simulink model "modelReferenceTest"  (Simulink 7.6)
settings: Solver=FixedStepDiscrete  StartTime=0.0  StopTime=10.0  FixedStep=1  RelTol=1e-3
settings Model: Creator=c2wt  LastModifiedBy=c2wt

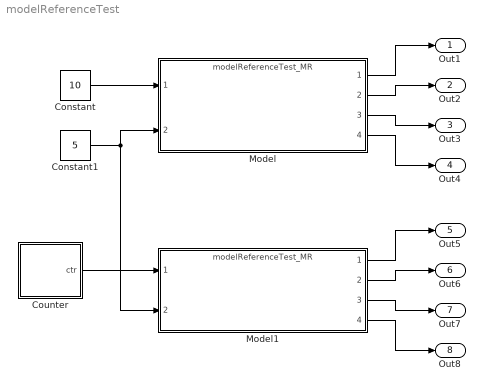
== system modelReferenceTest ==
  Constant : Constant  Value=10
  Constant1 : Constant  Value=5
  Counter : Stateflow chart  TreatAsAtomicUnit=on
  Model : ModelReference  ModelNameDialog=modelReferenceTest_MR  SimulationMode=Accelerator  ModelReferenceVersion=1.4  CopyOfModelName=modelReferenceTest_MR
  Model1 : ModelReference  ModelNameDialog=modelReferenceTest_MR  SimulationMode=Accelerator  ModelReferenceVersion=1.4  CopyOfModelName=modelReferenceTest_MR
  Out1 : Outport
  Out2 : Outport  Port=2
  Out3 : Outport  Port=3
  Out4 : Outport  Port=4
  Out5 : Outport  Port=5
  Out6 : Outport  Port=6
  Out7 : Outport  Port=7
  Out8 : Outport  Port=8
  wires:
  Constant/1 -> Model/1
  Constant1/1 -> Model/2, Model1/2
  Model/1 -> Out1/1
  Model/2 -> Out2/1
  Model/3 -> Out3/1
  Model/4 -> Out4/1
  Model1/1 -> Out5/1
  Model1/2 -> Out6/1
  Model1/3 -> Out7/1
  Model1/4 -> Out8/1
  Counter/1(ctr) -> Model1/1

== stateflow chart Counter ==
  state s1
  (default) -> s1
  s1 -> s1 [order 1] : [ctr < 4] / ctr = ctr+1;
  s1 -> s1 [order 2] : [ctr >= 4] / ctr = -2;
  data: ctr output double =1
